simulink model "Demo1sim"  (R2019a)
settings: Solver=VariableStepAuto  StartTime=0.0  StopTime=10.0  RelTol=1e-3
undefined symbols (not defined in the file): K_phi, K_rho, sigma_phi, sigma_rho
settings Model: Creator=hspol  LastModifiedBy=hspol

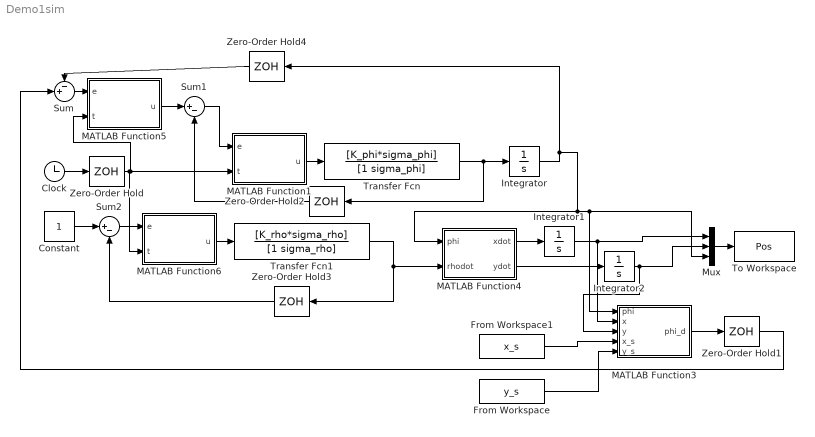
== system Demo1sim ==
  Clock : Clock
  Constant : Constant
  From Workspace : FromWorkspace  VariableName=y_s  SampleTime=0
  From Workspace1 : FromWorkspace  VariableName=x_s  SampleTime=0
  Integrator : Integrator
  Integrator1 : Integrator
  Integrator2 : Integrator
  MATLAB Function1 : MATLAB Function  TreatAsAtomicUnit=on
  MATLAB Function3 : MATLAB Function  TreatAsAtomicUnit=on
  MATLAB Function4 : MATLAB Function  TreatAsAtomicUnit=on
  MATLAB Function5 : MATLAB Function  TreatAsAtomicUnit=on
  MATLAB Function6 : MATLAB Function  TreatAsAtomicUnit=on
  Mux : Mux  Inputs=3
  Sum : Sum  Inputs=-+|
  Sum1 : Sum  Inputs=|+-
  Sum2 : Sum  Inputs=|+-
  To Workspace : ToWorkspace  VariableName=Pos  SaveFormat=Timeseries  SampleTime=-1
  Transfer Fcn : TransferFcn  Numerator=[K_phi*sigma_phi]  Denominator=[1 sigma_phi]
  Transfer Fcn1 : TransferFcn  Numerator=[K_rho*sigma_rho]  Denominator=[1 sigma_rho]
  Zero-Order Hold{,1..4} (5 alike) : ZeroOrderHold  SampleTime=-1
  wires:
  MATLAB Function5/1(u) -> Sum1/1
  Clock/1 -> Zero-Order Hold/1
  Zero-Order Hold/1 -> MATLAB Function6/2(t), MATLAB Function5/2(t), MATLAB Function1/2(t)
  Sum1/1 -> MATLAB Function1/1(e)
  Sum/1 -> MATLAB Function5/1(e)
  Zero-Order Hold4/1 -> Sum/1
  MATLAB Function1/1(u) -> Transfer Fcn/1
  Constant/1 -> Sum2/1
  Sum2/1 -> MATLAB Function6/1(e)
  MATLAB Function6/1(u) -> Transfer Fcn1/1
  Transfer Fcn1/1 -> MATLAB Function4/2(rhodot), Zero-Order Hold3/1
  Zero-Order Hold3/1 -> Sum2/2
  Transfer Fcn/1 -> Integrator/1, Zero-Order Hold2/1
  Zero-Order Hold2/1 -> Sum1/2
  Integrator/1 -> MATLAB Function3/1(phi), Mux/3, MATLAB Function4/1(phi), Zero-Order Hold4/1
  MATLAB Function4/1(xdot) -> Integrator1/1
  MATLAB Function4/2(ydot) -> Integrator2/1
  Integrator1/1 -> Mux/1, MATLAB Function3/2(x)
  Integrator2/1 -> MATLAB Function3/3(y), Mux/2
  Mux/1 -> To Workspace/1
  From Workspace1/1 -> MATLAB Function3/4(x_s)
  From Workspace/1 -> MATLAB Function3/5(y_s)
  MATLAB Function3/1(phi_d) -> Zero-Order Hold1/1
  Zero-Order Hold1/1 -> Sum/2

== matlab function Demo1sim/MATLAB Function1 ==
  data: e input; u output; t input
function u = fcn(e,t)

u = e * t;

== matlab function Demo1sim/MATLAB Function5 ==
  data: e input; u output; t input
function u = fcn(e,t)

u = e * t;

== matlab function Demo1sim/MATLAB Function3 ==
  data: phi input; phi_d output; x input; y input; x_s input; y_s input
function phi_d = fcn(phi,x,y,x_s,y_s)

phi_d = phi + atan2(y_s-y,x_s-x) - phi;

== matlab function Demo1sim/MATLAB Function4 ==
  data: phi input; xdot output; rhodot input; ydot output
function [xdot,ydot] = fcn(phi,rhodot)

xdot = rhodot*cos(phi);
ydot = rhotdot*sin(phi);

== matlab function Demo1sim/MATLAB Function6 ==
  data: e input; u output; t input
function u = fcn(e,t)

u = e * t;
